simulink model "PiSimulink_MCU"  (R2020b)
settings: Solver=FixedStepDiscrete  StartTime=0.0  StopTime=10.0  FixedStep=0.001  RelTol=1e-3  EnableMultiTasking=on
InitFcn:
  | mbd_s32k_consistency_checks(bdroot(gcs));
undefined symbols (not defined in the file): LQFP
libraries: mbd_s32k1xx_ec_toolbox x13, simulink x2
(part 1 of 2)
Description:
  | This code is the MCU half of the Simulink on Raspberry Pi Guide.
  | It determines the data that is sent from the MCU.
  | 
  | Extra Modules (In addition to default functions):
  | LPSPI1 (Pi SPI logic moved from defaults to user area)
  | 
  | For more information, see our Simulink on Raspberry Pi Guide:
  | https://www.audesseinc.com/labs/resources/simulinkmpu/
  | 
  | Revision: 1.3
settings Model: LastModifiedBy=prasa
settings DataIOCC: ExternalInput=off  InitialState=off  SaveOutput=off  SignalLogging=off  SaveTime=off
settings OptimizationCC: DefaultParameterBehavior=Inlined  DefaultUnderspecifiedDataType=single  EnhancedBackFolding=on  PassReuseOutputArgsAs=Individual arguments  OptimizeBlockOrder=speed  EfficientTunableParamExpr=on
settings DebuggingCC: InheritedTsInSrcMsg=none  SingleTaskRateTransMsg=error  ParameterTunabilityLossMsg=error  UnconnectedInputMsg=error  UnconnectedOutputMsg=error  UnconnectedLineMsg=error  UnknownTsInhSupMsg=error  ArithmeticOperatorsInVariantConditions=warning
settings HardwareCC: ProdBitPerPointer=32  ProdBitPerSizeT=32  ProdBitPerPtrDiffT=32  ProdLargestAtomicInteger=Long  ProdLargestAtomicFloat=Double  ProdWordSize=32  ProdHWDeviceType=ARM Compatible->ARM Cortex
settings SFSimCC: MATLABDynamicMemAlloc=off  CustomCodeUndefinedFunction=UseInterfaceOnly
settings RTWCC: Description=Model Based Design Toolbox S32K1xx Code Generation Target  SystemTargetFile=mbd_s32k.tlc  MakeCommand=mbd_s32k_make_rtw COPY_MDLREF_INCLUDES=0  TemplateMakefile=mbd_s32k.tmf  GenerateReport=on  IncludeHyperlinkInReport=on  LaunchReport=on  GenerateTraceInfo=on  GenerateTraceReport=on  GenerateTraceReportSl=on  GenerateTraceReportSf=on  GenerateTraceReportEml=on
settings CodeAppCC: ForceParamTrailComments=on  IgnoreCustomStorageClasses=off  OperatorAnnotations=on  SimulinkDataObjDesc=on  SFDataObjDesc=on  InsertBlockDesc=on  StateflowObjectComments=on
settings STFCustomTargetCC: TargetLangStandard=C99 (ISO)  MultiwordLength=256  ConcurrentExecutionCompliant=off  CombineOutputUpdateFcns=on  ERTCustomFileBanners=on  SupportContinuousTime=off  SupportNonInlinedSFcns=off  RemoveResetFunc=on  MATLABClassNameForMDSCustomization=Simulink.SoftwareTarget.ERTCustomization  CPPClassGenCompliant=off  GRTInterface=off  SystemTargetFile=mbd_s32k.tlc
settings ERTTargetCC: TargetLangStandard=C99 (ISO)  ParMdlRefBuildCompliant=off  CompOptLevelCompliant=off  ConcurrentExecutionCompliant=off  ModelStepFunctionPrototypeControlCompliant=off  CPPClassGenCompliant=off  UseToolchainInfoCompliant=off  InlinedParameterPlacement=NonHierarchical  ERTSrcFileBannerTemplate=mbd_ert_code_template.cgt  ERTHdrFileBannerTemplate=mbd_ert_code_template.cgt  ERTDataSrcFileTemplate=mbd_ert_code_template.cgt  ERTDataHdrFileTemplate=mbd_ert_code_template.cgt  ERTCustomFileTemplate=example_file_process.tlc

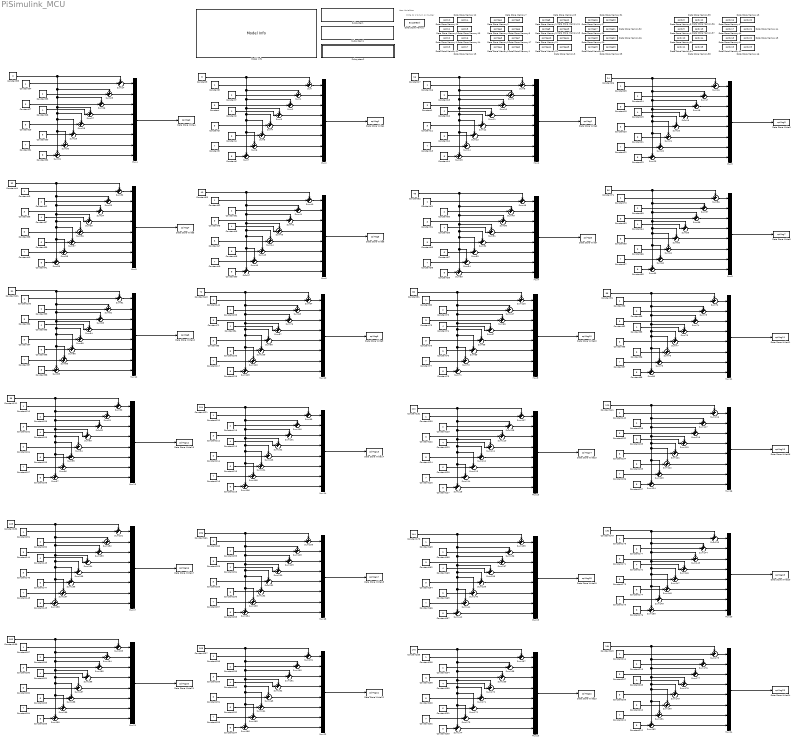
== system PiSimulink_MCU ==
  note: User Variables
  note: Write to 1 to turn on buzzer
  Constant{,1,18,27,36,45,54,63,72..73,82,92,102,112,122,132,144,153,162,171,180,189,198,207} (24 alike) : Constant  Value=3  OutDataTypeStr=uint8
  Constant{2,10,19,28,37,46,55,64,74,83..84,93,103,113,123,133,145,154,163,172,181,190,199,208} (24 alike) : Constant  Value=4  OutDataTypeStr=uint8
  Constant{8,16,25,34,43,52,61,70,80,90,100,110,120,130,140,142,151,160,169,178,187,196,205,214} (24 alike) : Constant  OutDataTypeStr=uint8
  Constant101 : Constant  Value=64  OutDataTypeStr=uint8
  Constant{3,11,20,29,38,47,56,65,75,85,94..95,104,114,124,134,146,155,164,173,182,191,200,209} (24 alike) : Constant  Value=5  OutDataTypeStr=uint8
  Constant{4,12,21,30,39,48,57,66,76,86,96,105..106,115,125,135,147,156,165,174,183,192,201,210} (24 alike) : Constant  Value=6  OutDataTypeStr=uint8
  Constant{5,13,22,31,40,49,58,67,77,87,97,107,116..117,126,136,148,157,166,175,184,193,202,211} (24 alike) : Constant  Value=7  OutDataTypeStr=uint8
  Constant{6,9,14,23,32,41,50,59,68,78,88,98,108,118,127..128,137,149,158,167,176,185,194,203,212} (25 alike) : Constant  Value=8  OutDataTypeStr=uint8
  Constant{7,15,24,33,42,51,60,69,79,89,99,109,119,129,138..139,150,159,168,177,186,195,204,213} (24 alike) : Constant  Value=2  OutDataTypeStr=uint8
  Constant111 : Constant  Value=96  OutDataTypeStr=uint8
  Constant121 : Constant  Value=104  OutDataTypeStr=uint8
  Constant131 : Constant  Value=112  OutDataTypeStr=uint8
  Constant141 : Constant  Value=120  OutDataTypeStr=uint8
  Constant143 : Constant  Value=72  OutDataTypeStr=uint8
  Constant152 : Constant  Value=128  OutDataTypeStr=uint8
  Constant161 : Constant  Value=136  OutDataTypeStr=uint8
  Constant17 : Constant  Value=16  OutDataTypeStr=uint8
  Constant170 : Constant  Value=144  OutDataTypeStr=uint8
  Constant179 : Constant  Value=152  OutDataTypeStr=uint8
  Constant188 : Constant  Value=160  OutDataTypeStr=uint8
  Constant197 : Constant  Value=168  OutDataTypeStr=uint8
  Constant206 : Constant  Value=176  OutDataTypeStr=uint8
  Constant215 : Constant  Value=184  OutDataTypeStr=uint8
  Constant26 : Constant  Value=24  OutDataTypeStr=uint8
  Constant35 : Constant  Value=0  OutDataTypeStr=uint8
  Constant44 : Constant  Value=32  OutDataTypeStr=uint8
  Constant53 : Constant  Value=40  OutDataTypeStr=uint8
  Constant62 : Constant  Value=48  OutDataTypeStr=uint8
  Constant71 : Constant  Value=56  OutDataTypeStr=uint8
  Constant81 : Constant  Value=80  OutDataTypeStr=uint8
  Constant91 : Constant  Value=88  OutDataTypeStr=uint8
  Data Store Memory : DataStoreMemory  DataStoreName=BuzzerBool  ReadBeforeWriteMsg=warning  WriteAfterWriteMsg=warning  WriteAfterReadMsg=warning  ShowAdditionalParam=off  OutDataTypeStr=boolean
  Data Store Memory1 : DataStoreMemory  DataStoreName=spiMsg0  ReadBeforeWriteMsg=warning  WriteAfterWriteMsg=warning  WriteAfterReadMsg=warning  InitialValue=[255 255 255 255 255 255 255 255]  ShowAdditionalParam=off  OutDataTypeStr=uint8
  Data Store Memory10 : DataStoreMemory  DataStoreName=spiRx2  ReadBeforeWriteMsg=warning  WriteAfterWriteMsg=warning  WriteAfterReadMsg=warning  InitialValue=[255 255 255 255 255 255 255 255]  ShowAdditionalParam=off  OutDataTypeStr=uint8
  Data Store Memory11 : DataStoreMemory  DataStoreName=spiRx3  ReadBeforeWriteMsg=warning  WriteAfterWriteMsg=warning  WriteAfterReadMsg=warning  InitialValue=[255 255 255 255 255 255 255 255]  ShowAdditionalParam=off  OutDataTypeStr=uint8
  Data Store Memory12 : DataStoreMemory  DataStoreName=spiRx4  ReadBeforeWriteMsg=warning  WriteAfterWriteMsg=warning  WriteAfterReadMsg=warning  InitialValue=[255 255 255 255 255 255 255 255]  ShowAdditionalParam=off  OutDataTypeStr=uint8
  Data Store Memory13 : DataStoreMemory  DataStoreName=spiRx5  ReadBeforeWriteMsg=warning  WriteAfterWriteMsg=warning  WriteAfterReadMsg=warning  InitialValue=[255 255 255 255 255 255 255 255]  ShowAdditionalParam=off  OutDataTypeStr=uint8
  Data Store Memory14 : DataStoreMemory  DataStoreName=spiRx6  ReadBeforeWriteMsg=warning  WriteAfterWriteMsg=warning  WriteAfterReadMsg=warning  InitialValue=[255 255 255 255 255 255 255 255]  ShowAdditionalParam=off  OutDataTypeStr=uint8
  Data Store Memory15 : DataStoreMemory  DataStoreName=spiRx7  ReadBeforeWriteMsg=warning  WriteAfterWriteMsg=warning  WriteAfterReadMsg=warning  InitialValue=[255 255 255 255 255 255 255 255]  ShowAdditionalParam=off  OutDataTypeStr=uint8
  Data Store Memory16 : DataStoreMemory  DataStoreName=spiRx0  ReadBeforeWriteMsg=warning  WriteAfterWriteMsg=warning  WriteAfterReadMsg=warning  InitialValue=[255 255 255 255 255 255 255 255]  ShowAdditionalParam=off  OutDataTypeStr=uint8
  Data Store Memory17 : DataStoreMemory  DataStoreName=spiMsg7  ReadBeforeWriteMsg=warning  WriteAfterWriteMsg=warning  WriteAfterReadMsg=warning  InitialValue=[255 255 255 255 255 255 255 255]  ShowAdditionalParam=off  OutDataTypeStr=uint8
  Data Store Memory18 : DataStoreMemory  DataStoreName=spiMsg14  ReadBeforeWriteMsg=warning  WriteAfterWriteMsg=warning  WriteAfterReadMsg=warning  InitialValue=[255 255 255 255 255 255 255 255]  ShowAdditionalParam=off  OutDataTypeStr=uint8
  Data Store Memory19 : DataStoreMemory  DataStoreName=spiMsg8  ReadBeforeWriteMsg=warning  WriteAfterWriteMsg=warning  WriteAfterReadMsg=warning  InitialValue=[255 255 255 255 255 255 255 255]  ShowAdditionalParam=off  OutDataTypeStr=uint8
  Data Store Memory2 : DataStoreMemory  DataStoreName=spiMsg1  ReadBeforeWriteMsg=warning  WriteAfterWriteMsg=warning  WriteAfterReadMsg=warning  InitialValue=[255 255 255 255 255 255 255 255]  ShowAdditionalParam=off  OutDataTypeStr=uint8
  Data Store Memory20 : DataStoreMemory  DataStoreName=spiMsg9  ReadBeforeWriteMsg=warning  WriteAfterWriteMsg=warning  WriteAfterReadMsg=warning  InitialValue=[255 255 255 255 255 255 255 255]  ShowAdditionalParam=off  OutDataTypeStr=uint8
  Data Store Memory21 : DataStoreMemory  DataStoreName=spiMsg10  ReadBeforeWriteMsg=warning  WriteAfterWriteMsg=warning  WriteAfterReadMsg=warning  InitialValue=[255 255 255 255 255 255 255 255]  ShowAdditionalParam=off  OutDataTypeStr=uint8
  Data Store Memory22 : DataStoreMemory  DataStoreName=spiMsg11  ReadBeforeWriteMsg=warning  WriteAfterWriteMsg=warning  WriteAfterReadMsg=warning  InitialValue=[255 255 255 255 255 255 255 255]  ShowAdditionalParam=off  OutDataTypeStr=uint8
  Data Store Memory23 : DataStoreMemory  DataStoreName=spiMsg12  ReadBeforeWriteMsg=warning  WriteAfterWriteMsg=warning  WriteAfterReadMsg=warning  InitialValue=[255 255 255 255 255 255 255 255]  ShowAdditionalParam=off  OutDataTypeStr=uint8
  Data Store Memory24 : DataStoreMemory  DataStoreName=spiMsg13  ReadBeforeWriteMsg=warning  WriteAfterWriteMsg=warning  WriteAfterReadMsg=warning  InitialValue=[255 255 255 255 255 255 255 255]  ShowAdditionalParam=off  OutDataTypeStr=uint8
  Data Store Memory25 : DataStoreMemory  DataStoreName=spiMsg23  ReadBeforeWriteMsg=warning  WriteAfterWriteMsg=warning  WriteAfterReadMsg=warning  InitialValue=[255 255 255 255 255 255 255 255]  ShowAdditionalParam=off  OutDataTypeStr=uint8
  Data Store Memory26 : DataStoreMemory  DataStoreName=spiMsg22  ReadBeforeWriteMsg=warning  WriteAfterWriteMsg=warning  WriteAfterReadMsg=warning  InitialValue=[255 255 255 255 255 255 255 255]  ShowAdditionalParam=off  OutDataTypeStr=uint8
  Data Store Memory27 : DataStoreMemory  DataStoreName=spiMsg16  ReadBeforeWriteMsg=warning  WriteAfterWriteMsg=warning  WriteAfterReadMsg=warning  InitialValue=[255 255 255 255 255 255 255 255]  ShowAdditionalParam=off  OutDataTypeStr=uint8
  Data Store Memory28 : DataStoreMemory  DataStoreName=spiMsg17  ReadBeforeWriteMsg=warning  WriteAfterWriteMsg=warning  WriteAfterReadMsg=warning  InitialValue=[255 255 255 255 255 255 255 255]  ShowAdditionalParam=off  OutDataTypeStr=uint8
  Data Store Memory29 : DataStoreMemory  DataStoreName=spiMsg18  ReadBeforeWriteMsg=warning  WriteAfterWriteMsg=warning  WriteAfterReadMsg=warning  InitialValue=[255 255 255 255 255 255 255 255]  ShowAdditionalParam=off  OutDataTypeStr=uint8
  Data Store Memory3 : DataStoreMemory  DataStoreName=spiMsg15  ReadBeforeWriteMsg=warning  WriteAfterWriteMsg=warning  WriteAfterReadMsg=warning  InitialValue=[255 255 255 255 255 255 255 255]  ShowAdditionalParam=off  OutDataTypeStr=uint8
  Data Store Memory30 : DataStoreMemory  DataStoreName=spiMsg19  ReadBeforeWriteMsg=warning  WriteAfterWriteMsg=warning  WriteAfterReadMsg=warning  InitialValue=[255 255 255 255 255 255 255 255]  ShowAdditionalParam=off  OutDataTypeStr=uint8
  Data Store Memory31 : DataStoreMemory  DataStoreName=spiMsg20  ReadBeforeWriteMsg=warning  WriteAfterWriteMsg=warning  WriteAfterReadMsg=warning  InitialValue=[255 255 255 255 255 255 255 255]  ShowAdditionalParam=off  OutDataTypeStr=uint8
  Data Store Memory32 : DataStoreMemory  DataStoreName=spiMsg21  ReadBeforeWriteMsg=warning  WriteAfterWriteMsg=warning  WriteAfterReadMsg=warning  InitialValue=[255 255 255 255 255 255 255 255]  ShowAdditionalParam=off  OutDataTypeStr=uint8
  Data Store Memory33 : DataStoreMemory  DataStoreName=spiRx10  ReadBeforeWriteMsg=warning  WriteAfterWriteMsg=warning  WriteAfterReadMsg=warning  InitialValue=[255 255 255 255 255 255 255 255]  ShowAdditionalParam=off  OutDataTypeStr=uint8
  Data Store Memory34 : DataStoreMemory  DataStoreName=spiRx11  ReadBeforeWriteMsg=warning  WriteAfterWriteMsg=warning  WriteAfterReadMsg=warning  InitialValue=[255 255 255 255 255 255 255 255]  ShowAdditionalParam=off  OutDataTypeStr=uint8
  Data Store Memory35 : DataStoreMemory  DataStoreName=spiRx12  ReadBeforeWriteMsg=warning  WriteAfterWriteMsg=warning  WriteAfterReadMsg=warning  InitialValue=[255 255 255 255 255 255 255 255]  ShowAdditionalParam=off  OutDataTypeStr=uint8
  Data Store Memory36 : DataStoreMemory  DataStoreName=spiRx13  ReadBeforeWriteMsg=warning  WriteAfterWriteMsg=warning  WriteAfterReadMsg=warning  InitialValue=[255 255 255 255 255 255 255 255]  ShowAdditionalParam=off  OutDataTypeStr=uint8
  Data Store Memory37 : DataStoreMemory  DataStoreName=spiRx14  ReadBeforeWriteMsg=warning  WriteAfterWriteMsg=warning  WriteAfterReadMsg=warning  InitialValue=[255 255 255 255 255 255 255 255]  ShowAdditionalParam=off  OutDataTypeStr=uint8
  Data Store Memory38 : DataStoreMemory  DataStoreName=spiRx15  ReadBeforeWriteMsg=warning  WriteAfterWriteMsg=warning  WriteAfterReadMsg=warning  InitialValue=[255 255 255 255 255 255 255 255]  ShowAdditionalParam=off  OutDataTypeStr=uint8
  Data Store Memory39 : DataStoreMemory  DataStoreName=spiRx8  ReadBeforeWriteMsg=warning  WriteAfterWriteMsg=warning  WriteAfterReadMsg=warning  InitialValue=[255 255 255 255 255 255 255 255]  ShowAdditionalParam=off  OutDataTypeStr=uint8
  Data Store Memory4 : DataStoreMemory  DataStoreName=spiMsg2  ReadBeforeWriteMsg=warning  WriteAfterWriteMsg=warning  WriteAfterReadMsg=warning  InitialValue=[255 255 255 255 255 255 255 255]  ShowAdditionalParam=off  OutDataTypeStr=uint8
  Data Store Memory40 : DataStoreMemory  DataStoreName=spiRx9  ReadBeforeWriteMsg=warning  WriteAfterWriteMsg=warning  WriteAfterReadMsg=warning  InitialValue=[255 255 255 255 255 255 255 255]  ShowAdditionalParam=off  OutDataTypeStr=uint8
  Data Store Memory41 : DataStoreMemory  DataStoreName=spiRx18  ReadBeforeWriteMsg=warning  WriteAfterWriteMsg=warning  WriteAfterReadMsg=warning  InitialValue=[255 255 255 255 255 255 255 255]  ShowAdditionalParam=off  OutDataTypeStr=uint8
  Data Store Memory42 : DataStoreMemory  DataStoreName=spiRx19  ReadBeforeWriteMsg=warning  WriteAfterWriteMsg=warning  WriteAfterReadMsg=warning  InitialValue=[255 255 255 255 255 255 255 255]  ShowAdditionalParam=off  OutDataTypeStr=uint8
  Data Store Memory43 : DataStoreMemory  DataStoreName=spiRx20  ReadBeforeWriteMsg=warning  WriteAfterWriteMsg=warning  WriteAfterReadMsg=warning  InitialValue=[255 255 255 255 255 255 255 255]  ShowAdditionalParam=off  OutDataTypeStr=uint8
  Data Store Memory44 : DataStoreMemory  DataStoreName=spiRx21  ReadBeforeWriteMsg=warning  WriteAfterWriteMsg=warning  WriteAfterReadMsg=warning  InitialValue=[255 255 255 255 255 255 255 255]  ShowAdditionalParam=off  OutDataTypeStr=uint8
  Data Store Memory45 : DataStoreMemory  DataStoreName=spiRx22  ReadBeforeWriteMsg=warning  WriteAfterWriteMsg=warning  WriteAfterReadMsg=warning  InitialValue=[255 255 255 255 255 255 255 255]  ShowAdditionalParam=off  OutDataTypeStr=uint8
  Data Store Memory46 : DataStoreMemory  DataStoreName=spiRx23  ReadBeforeWriteMsg=warning  WriteAfterWriteMsg=warning  WriteAfterReadMsg=warning  InitialValue=[255 255 255 255 255 255 255 255]  ShowAdditionalParam=off  OutDataTypeStr=uint8
  Data Store Memory47 : DataStoreMemory  DataStoreName=spiRx16  ReadBeforeWriteMsg=warning  WriteAfterWriteMsg=warning  WriteAfterReadMsg=warning  InitialValue=[255 255 255 255 255 255 255 255]  ShowAdditionalParam=off  OutDataTypeStr=uint8
  Data Store Memory48 : DataStoreMemory  DataStoreName=spiRx17  ReadBeforeWriteMsg=warning  WriteAfterWriteMsg=warning  WriteAfterReadMsg=warning  InitialValue=[255 255 255 255 255 255 255 255]  ShowAdditionalParam=off  OutDataTypeStr=uint8
  Data Store Memory5 : DataStoreMemory  DataStoreName=spiMsg3  ReadBeforeWriteMsg=warning  WriteAfterWriteMsg=warning  WriteAfterReadMsg=warning  InitialValue=[255 255 255 255 255 255 255 255]  ShowAdditionalParam=off  OutDataTypeStr=uint8
  Data Store Memory6 : DataStoreMemory  DataStoreName=spiMsg4  ReadBeforeWriteMsg=warning  WriteAfterWriteMsg=warning  WriteAfterReadMsg=warning  InitialValue=[255 255 255 255 255 255 255 255]  ShowAdditionalParam=off  OutDataTypeStr=uint8
  Data Store Memory7 : DataStoreMemory  DataStoreName=spiMsg5  ReadBeforeWriteMsg=warning  WriteAfterWriteMsg=warning  WriteAfterReadMsg=warning  InitialValue=[255 255 255 255 255 255 255 255]  ShowAdditionalParam=off  OutDataTypeStr=uint8
  Data Store Memory8 : DataStoreMemory  DataStoreName=spiMsg6  ReadBeforeWriteMsg=warning  WriteAfterWriteMsg=warning  WriteAfterReadMsg=warning  InitialValue=[255 255 255 255 255 255 255 255]  ShowAdditionalParam=off  OutDataTypeStr=uint8
  Data Store Memory9 : DataStoreMemory  DataStoreName=spiRx1  ReadBeforeWriteMsg=warning  WriteAfterWriteMsg=warning  WriteAfterReadMsg=warning  InitialValue=[255 255 255 255 255 255 255 255]  ShowAdditionalParam=off  OutDataTypeStr=uint8
  Data Store Write1 : DataStoreWrite  DataStoreName=spiMsg1
  Data Store Write10 : DataStoreWrite  DataStoreName=spiMsg10
  Data Store Write11 : DataStoreWrite  DataStoreName=spiMsg11
  Data Store Write12 : DataStoreWrite  DataStoreName=spiMsg8
  Data Store Write13 : DataStoreWrite  DataStoreName=spiMsg12
  Data Store Write14 : DataStoreWrite  DataStoreName=spiMsg13
  Data Store Write15 : DataStoreWrite  DataStoreName=spiMsg14
  Data Store Write16 : DataStoreWrite  DataStoreName=spiMsg15
  Data Store Write17 : DataStoreWrite  DataStoreName=spiMsg16
  Data Store Write18 : DataStoreWrite  DataStoreName=spiMsg17
  Data Store Write19 : DataStoreWrite  DataStoreName=spiMsg18
  Data Store Write2 : DataStoreWrite  DataStoreName=spiMsg2
  Data Store Write20 : DataStoreWrite  DataStoreName=spiMsg19
  Data Store Write21 : DataStoreWrite  DataStoreName=spiMsg20
  Data Store Write22 : DataStoreWrite  DataStoreName=spiMsg21
  Data Store Write23 : DataStoreWrite  DataStoreName=spiMsg22
  Data Store Write24 : DataStoreWrite  DataStoreName=spiMsg23
  Data Store Write3 : DataStoreWrite  DataStoreName=spiMsg3
  Data Store Write4 : DataStoreWrite  DataStoreName=spiMsg0
  Data Store Write5 : DataStoreWrite  DataStoreName=spiMsg4
  Data Store Write6 : DataStoreWrite  DataStoreName=spiMsg5
  Data Store Write7 : DataStoreWrite  DataStoreName=spiMsg6
  Data Store Write8 : DataStoreWrite  DataStoreName=spiMsg7
  Data Store Write9 : DataStoreWrite  DataStoreName=spiMsg9
  Model Info : simulink/Model-Wide Utilities/Model Info  Frame=on  DisplayStringWithTags=|  HorizontalTextAlignment=Left  LeftAlignmentValue=0.02
      | Audesse Simulink Samples: %<ModelName>
      | 
      | %<Description>
  Mux{1..24} (24 alike) : Mux  Inputs=8
  Subsystem : Subsystem  Priority=1
      mask Display:
      | scl=1/4;
      | patch(scl*[0,52,90,54],scl*[16,55,146,146],[16/255,118/255,188/255],'bottom-left');
      | patch(scl*[0,27,82,77,68],scl*[16,0,42,62,69],[46/255,49/255,146/255],'bottom-left');
      | patch(scl*[89,125,90,68],scl*[16,16,146,91],[0,0,0],'bottom-left');
      | disp('Hardware Modules Config\n(SPI,CAN,ADC,etc..)');
  Subsystem1 : Subsystem
      mask Display:
      | scl=1/4;
      | patch(scl*[0,52,90,54],scl*[16,55,146,146],[16/255,118/255,188/255],'bottom-left');
      | patch(scl*[0,27,82,77,68],scl*[16,0,42,62,69],[46/255,49/255,146/255],'bottom-left');
      | patch(scl*[89,125,90,68],scl*[16,16,146,91],[0,0,0],'bottom-left');
      | disp('Default Control Functions\n(Do not modify unless you know what you are doing)');
  Subsystem2 : Subsystem
      mask Display:
      | scl=1/4;
      | patch(scl*[0,52,90,54],scl*[16,55,146,146],[16/255,118/255,188/255],'bottom-left');
      | patch(scl*[0,27,82,77,68],scl*[16,0,42,62,69],[46/255,49/255,146/255],'bottom-left');
      | patch(scl*[89,125,90,68],scl*[16,16,146,91],[0,0,0],'bottom-left');
      | disp('Run Once at Startup');
  Sum{,1..191} (192 alike) : Sum  Inputs=++|
  wires:
  Mux2/1 -> Data Store Write1/1
  Sum/1 -> Mux2/1
  Sum1/1 -> Mux2/2
  Sum2/1 -> Mux2/3
  Sum3/1 -> Mux2/4
  Sum4/1 -> Mux2/5
  Sum7/1 -> Mux2/8
  Sum6/1 -> Mux2/7
  Sum5/1 -> Mux2/6
  Constant6/1 -> Sum7/2
  Constant5/1 -> Sum6/2
  Constant4/1 -> Sum5/2
  Constant3/1 -> Sum4/2
  Constant2/1 -> Sum3/2
  Constant/1 -> Sum2/2
  Constant7/1 -> Sum1/2
  Constant8/1 -> Sum/2
  Constant9/1 -> Sum1/1, Sum2/1, Sum3/1, Sum4/1, Sum7/1, Sum6/1, Sum5/1, Sum/1
  Sum9/1 -> Mux1/2
  Sum8/1 -> Mux1/1
  Sum14/1 -> Mux1/7
  Constant15/1 -> Sum9/2
  Constant11/1 -> Sum12/2
  Constant10/1 -> Sum11/2
  Constant12/1 -> Sum13/2
  Constant16/1 -> Sum8/2
  Sum10/1 -> Mux1/3
  Sum11/1 -> Mux1/4
  Sum13/1 -> Mux1/6
  Constant14/1 -> Sum15/2
  Sum15/1 -> Mux1/8
  Mux1/1 -> Data Store Write2/1
  Constant17/1 -> Sum9/1, Sum10/1, Sum11/1, Sum12/1, Sum15/1, Sum14/1, Sum13/1, Sum8/1
  Constant1/1 -> Sum10/2
  Sum12/1 -> Mux1/5
  Constant13/1 -> Sum14/2
  Sum17/1 -> Mux3/2
  Sum16/1 -> Mux3/1
  Sum22/1 -> Mux3/7
  Constant24/1 -> Sum17/2
  Constant20/1 -> Sum20/2
  Constant19/1 -> Sum19/2
  Constant21/1 -> Sum21/2
  Constant25/1 -> Sum16/2
  Sum18/1 -> Mux3/3
  Sum19/1 -> Mux3/4
  Sum21/1 -> Mux3/6
  Constant23/1 -> Sum23/2
  Sum23/1 -> Mux3/8
  Mux3/1 -> Data Store Write3/1
  Constant26/1 -> Sum17/1, Sum18/1, Sum19/1, Sum20/1, Sum23/1, Sum22/1, Sum21/1, Sum16/1
  Constant18/1 -> Sum18/2
  Sum20/1 -> Mux3/5
  Constant22/1 -> Sum22/2
  Sum25/1 -> Mux4/2
  Sum24/1 -> Mux4/1
  Sum30/1 -> Mux4/7
  Constant33/1 -> Sum25/2
  Constant29/1 -> Sum28/2
  Constant28/1 -> Sum27/2
  Constant30/1 -> Sum29/2
  Constant34/1 -> Sum24/2
  Sum26/1 -> Mux4/3
  Sum27/1 -> Mux4/4
  Sum29/1 -> Mux4/6
  Constant32/1 -> Sum31/2
  Sum31/1 -> Mux4/8
  Mux4/1 -> Data Store Write4/1
  Constant35/1 -> Sum25/1, Sum26/1, Sum27/1, Sum28/1, Sum31/1, Sum30/1, Sum29/1, Sum24/1
  Constant27/1 -> Sum26/2
  Sum28/1 -> Mux4/5
  Constant31/1 -> Sum30/2
  Sum33/1 -> Mux5/2
  Sum32/1 -> Mux5/1
  Sum38/1 -> Mux5/7
  Constant42/1 -> Sum33/2
  Constant38/1 -> Sum36/2
  Constant37/1 -> Sum35/2
  Constant39/1 -> Sum37/2
  Constant43/1 -> Sum32/2
  Sum34/1 -> Mux5/3
  Sum35/1 -> Mux5/4
  Sum37/1 -> Mux5/6
  Constant41/1 -> Sum39/2
  Sum39/1 -> Mux5/8
  Mux5/1 -> Data Store Write5/1
  Constant44/1 -> Sum33/1, Sum34/1, Sum35/1, Sum36/1, Sum39/1, Sum38/1, Sum37/1, Sum32/1
  Constant36/1 -> Sum34/2
  Sum36/1 -> Mux5/5
  Constant40/1 -> Sum38/2
  Sum41/1 -> Mux6/2
  Sum40/1 -> Mux6/1
  Sum46/1 -> Mux6/7
  Constant51/1 -> Sum41/2
  Constant47/1 -> Sum44/2
  Constant46/1 -> Sum43/2
  Constant48/1 -> Sum45/2
  Constant52/1 -> Sum40/2
  Sum42/1 -> Mux6/3
  Sum43/1 -> Mux6/4
  Sum45/1 -> Mux6/6
  Constant50/1 -> Sum47/2
  Sum47/1 -> Mux6/8
  Mux6/1 -> Data Store Write6/1
  Constant53/1 -> Sum41/1, Sum42/1, Sum43/1, Sum44/1, Sum47/1, Sum46/1, Sum45/1, Sum40/1
  Constant45/1 -> Sum42/2
  Sum44/1 -> Mux6/5
  Constant49/1 -> Sum46/2
  Sum49/1 -> Mux7/2
  Sum48/1 -> Mux7/1
  Sum54/1 -> Mux7/7
  Constant60/1 -> Sum49/2
  Constant56/1 -> Sum52/2
  Constant55/1 -> Sum51/2
  Constant57/1 -> Sum53/2
  Constant61/1 -> Sum48/2
  Sum50/1 -> Mux7/3
  Sum51/1 -> Mux7/4
  Sum53/1 -> Mux7/6
  Constant59/1 -> Sum55/2
  Sum55/1 -> Mux7/8
  Mux7/1 -> Data Store Write7/1
  Constant62/1 -> Sum49/1, Sum50/1, Sum51/1, Sum52/1, Sum55/1, Sum54/1, Sum53/1, Sum48/1
  Constant54/1 -> Sum50/2
  Sum52/1 -> Mux7/5
  Constant58/1 -> Sum54/2
  Sum57/1 -> Mux8/2
  Sum56/1 -> Mux8/1
  Sum62/1 -> Mux8/7
  Constant69/1 -> Sum57/2
  Constant65/1 -> Sum60/2
  Constant64/1 -> Sum59/2
  Constant66/1 -> Sum61/2
  Constant70/1 -> Sum56/2
  Sum58/1 -> Mux8/3
  Sum59/1 -> Mux8/4
  Sum61/1 -> Mux8/6
  Constant68/1 -> Sum63/2
  Sum63/1 -> Mux8/8
  Mux8/1 -> Data Store Write8/1
  Constant71/1 -> Sum57/1, Sum58/1, Sum59/1, Sum60/1, Sum63/1, Sum62/1, Sum61/1, Sum56/1
  Constant63/1 -> Sum58/2
  Sum60/1 -> Mux8/5
  Constant67/1 -> Sum62/2
  Constant81/1 -> Sum127/1, Sum66/1, Sum67/1, Sum68/1, Sum71/1, Sum70/1, Sum69/1, Sum126/1
  Constant73/1 -> Sum66/2
  Sum66/1 -> Mux9/3
  Sum71/1 -> Mux9/8
  Sum67/1 -> Mux9/4
  Constant75/1 -> Sum68/2
  Sum126/1 -> Mux9/1
  Constant76/1 -> Sum69/2
  Constant111/1 -> Sum91/1, Sum92/1, Sum93/1, Sum94/1, Sum97/1, Sum96/1, Sum95/1, Sum90/1
  Constant102/1 -> Sum92/2
  Sum94/1 -> Mux13/5
  Mux13/1 -> Data Store Write13/1
  Sum70/1 -> Mux9/7
  Sum97/1 -> Mux13/8
  Sum93/1 -> Mux13/4
  Constant105/1 -> Sum95/2
  Constant110/1 -> Sum90/2
  Constant103/1 -> Sum93/2
  Sum91/1 -> Mux13/2
  Sum96/1 -> Mux13/7
  Sum90/1 -> Mux13/1
  Constant109/1 -> Sum91/2
  Sum65/1 -> Mux10/2
  Constant133/1 -> Sum119/2
  Constant135/1 -> Sum122/2
  Constant134/1 -> Sum121/2
  Sum116/1 -> Mux16/1
  Constant138/1 -> Sum117/2
  Sum123/1 -> Mux16/7
  Sum117/1 -> Mux16/2
  Constant126/1 -> Sum114/2
  Constant136/1 -> Sum123/2
  Constant122/1 -> Sum110/2
  Constant79/1 -> Sum127/2
  Sum111/1 -> Mux15/4
  Sum121/1 -> Mux16/5
  Constant132/1 -> Sum118/2
  Sum115/1 -> Mux15/8
  Sum113/1 -> Mux15/6
  Constant127/1 -> Sum115/2
  Constant129/1 -> Sum108/2
  Sum107/1 -> Mux15/1
  Constant125/1 -> Sum113/2
  Constant124/1 -> Sum112/2
  Constant141/1 -> Sum117/1, Sum118/1, Sum119/1, Sum121/1, Sum124/1, Sum123/1, Sum122/1, Sum116/1
  Constant77/1 -> Sum70/2
  Sum114/1 -> Mux15/7
  Constant123/1 -> Sum111/2
  Sum68/1 -> Mux9/5
  Sum108/1 -> Mux15/2
  Mux16/1 -> Data Store Write16/1
  Constant104/1 -> Sum94/2
  Sum124/1 -> Mux16/8
  Constant137/1 -> Sum124/2
  Constant140/1 -> Sum116/2
  Sum118/1 -> Mux16/3
  Constant108/1 -> Sum97/2
  Sum119/1 -> Mux16/4
  Sum95/1 -> Mux13/6
  Sum73/1 -> Mux11/2
  Sum64/1 -> Mux10/1
  Constant116/1 -> Sum105/2
  Sum103/1 -> Mux14/5
  Sum92/1 -> Mux13/3
  Sum122/1 -> Mux16/6
  Constant121/1 -> Sum100/1, Sum101/1, Sum102/1, Sum103/1, Sum106/1, Sum105/1, Sum104/1, Sum99/1
  Constant112/1 -> Sum101/2
  Sum106/1 -> Mux14/8
  Constant118/1 -> Sum106/2
  Sum104/1 -> Mux14/6
  Constant131/1 -> Sum108/1, Sum110/1, Sum111/1, Sum112/1, Sum115/1, Sum114/1, Sum113/1, Sum107/1
  Sum102/1 -> Mux14/4
  Mux14/1 -> Data Store Write14/1
  Constant115/1 -> Sum104/2
  Constant78/1 -> Sum71/2
  Constant119/1 -> Sum100/2
  Sum101/1 -> Mux14/3
  Constant107/1 -> Sum96/2
  Constant120/1 -> Sum99/2
  Sum105/1 -> Mux14/7
  Sum100/1 -> Mux14/2
  Constant114/1 -> Sum103/2
  Constant113/1 -> Sum102/2
  Sum99/1 -> Mux14/1
  Sum120/1 -> Mux10/7
  Constant139/1 -> Sum65/2
  Constant87/1 -> Sum79/2
  Constant82/1 -> Sum74/2
  Sum77/1 -> Mux11/5
  Constant91/1 -> Sum73/1, Sum74/1, Sum75/1, Sum77/1, Sum80/1, Sum79/1, Sum78/1, Sum72/1
  Constant80/1 -> Sum126/2
  Mux11/1 -> Data Store Write11/1
  Sum75/1 -> Mux11/4
  Sum78/1 -> Mux11/6
  Constant88/1 -> Sum80/2
  Constant90/1 -> Sum72/2
  Constant89/1 -> Sum73/2
  Constant86/1 -> Sum78/2
  Sum72/1 -> Mux11/1
  Sum79/1 -> Mux11/7
  Constant130/1 -> Sum107/2
  Constant95/1 -> Sum98/2
  Constant84/1 -> Sum87/2
  Sum76/1 -> Mux10/3
  Sum87/1 -> Mux10/4
  Sum80/1 -> Mux11/8
  Constant97/1 -> Sum88/2
  Constant92/1 -> Sum83/2
  Sum85/1 -> Mux12/5
  Constant101/1 -> Sum82/1, Sum83/1, Sum84/1, Sum85/1, Sum89/1, Sum88/1, Sum86/1, Sum81/1
  Sum109/1 -> Mux10/6
  Mux15/1 -> Data Store Write15/1
  Sum69/1 -> Mux9/6
  Constant85/1 -> Sum77/2
  Constant74/1 -> Sum67/2
  Constant142/1 -> Sum64/2
  Sum83/1 -> Mux12/3
  Sum74/1 -> Mux11/3
  Mux12/1 -> Data Store Write12/1
  Sum86/1 -> Mux12/6
  Sum89/1 -> Mux12/8
  Constant93/1 -> Sum84/2
  Sum81/1 -> Mux12/1
  Constant96/1 -> Sum86/2
  Sum110/1 -> Mux15/3
  Constant106/1 -> Sum109/2
  Sum88/1 -> Mux12/7
  Constant99/1 -> Sum82/2
  Constant94/1 -> Sum85/2
  Sum112/1 -> Mux15/5
  Constant100/1 -> Sum81/2
  Constant83/1 -> Sum75/2
  Constant128/1 -> Sum125/2
  Sum84/1 -> Mux12/4
  Sum125/1 -> Mux10/8
  Sum127/1 -> Mux9/2
  Mux10/1 -> Data Store Write9/1
  Constant143/1 -> Sum65/1, Sum76/1, Sum87/1, Sum98/1, Sum125/1, Sum120/1, Sum109/1, Sum64/1
  Constant98/1 -> Sum89/2
  Mux9/1 -> Data Store Write10/1
  Sum82/1 -> Mux12/2
  Constant72/1 -> Sum76/2
  Sum98/1 -> Mux10/5
  Constant117/1 -> Sum120/2
  Constant164/1 -> Sum139/2
  Sum135/1 -> Mux19/1
  Constant165/1 -> Sum140/2
  Constant167/1 -> Sum142/2
  Sum140/1 -> Mux19/6
  Sum142/1 -> Mux19/8
  Constant171/1 -> Sum145/2
  Constant175/1 -> Sum149/2
  Constant162/1 -> Sum137/2
  Sum138/1 -> Mux19/4
  Sum147/1 -> Mux20/5
  Constant172/1 -> Sum146/2
  Sum149/1 -> Mux20/7
  Sum144/1 -> Mux20/2
  Sum143/1 -> Mux20/1
  Constant177/1 -> Sum144/2
  Constant173/1 -> Sum147/2
  Constant174/1 -> Sum148/2
  Constant166/1 -> Sum141/2
  Sum151/1 -> Mux17/1
  Constant150/1 -> Sum152/2
  Constant147/1 -> Sum156/2
  Constant151/1 -> Sum151/2
  Sum158/1 -> Mux17/8
  Sum157/1 -> Mux17/7
  Sum152/1 -> Mux17/2
  Constant168/1 -> Sum136/2
  Constant145/1 -> Sum154/2
  Mux17/1 -> Data Store Write17/1
  Sum155/1 -> Mux17/5
  Constant144/1 -> Sum153/2
  Constant152/1 -> Sum152/1, Sum153/1, Sum154/1, Sum155/1, Sum158/1, Sum157/1, Sum156/1, Sum151/1
  Constant158/1 -> Sum134/2
  Constant153/1 -> Sum129/2
  Sum132/1 -> Mux18/6
  Sum131/1 -> Mux18/5
  Constant157/1 -> Sum133/2
  Constant176/1 -> Sum150/2
  Sum150/1 -> Mux20/8
  Sum148/1 -> Mux20/6
  Sum136/1 -> Mux19/2
  Sum153/1 -> Mux17/3
  Sum141/1 -> Mux19/7
  Constant146/1 -> Sum155/2
  Constant161/1 -> Sum128/1, Sum129/1, Sum130/1, Sum131/1, Sum134/1, Sum133/1, Sum132/1, Sum159/1
  Mux20/1 -> Data Store Write20/1
  Sum145/1 -> Mux20/3
  Constant179/1 -> Sum144/1, Sum145/1, Sum146/1, Sum147/1, Sum150/1, Sum149/1, Sum148/1, Sum143/1
  Constant178/1 -> Sum143/2
  Sum156/1 -> Mux17/6
  Sum130/1 -> Mux18/4
  Mux18/1 -> Data Store Write18/1
  Constant156/1 -> Sum132/2
  Constant163/1 -> Sum138/2
  Sum154/1 -> Mux17/4
  Constant149/1 -> Sum158/2
  Sum139/1 -> Mux19/5
  Sum146/1 -> Mux20/4
  Sum137/1 -> Mux19/3
  Mux19/1 -> Data Store Write19/1
  Constant169/1 -> Sum135/2
  Sum159/1 -> Mux18/1
  Constant148/1 -> Sum157/2
  Sum129/1 -> Mux18/3
  Constant170/1 -> Sum136/1, Sum137/1, Sum138/1, Sum139/1, Sum142/1, Sum141/1, Sum140/1, Sum135/1
  Sum128/1 -> Mux18/2
  Constant159/1 -> Sum128/2
  Sum134/1 -> Mux18/8
  Constant160/1 -> Sum159/2
  Constant154/1 -> Sum130/2
  Sum133/1 -> Mux18/7
  Constant155/1 -> Sum131/2
  Sum167/1 -> Mux23/1
  Constant196/1 -> Sum191/2
  Sum166/1 -> Mux22/8
  Sum165/1 -> Mux22/7
  Constant191/1 -> Sum163/2
  Constant195/1 -> Sum160/2
  Constant190/1 -> Sum162/2
  Sum160/1 -> Mux22/2
  Sum161/1 -> Mux22/3
  Sum178/1 -> Mux24/4
  Mux23/1 -> Data Store Write23/1
  Sum169/1 -> Mux23/3
  Constant205/1 -> Sum167/2
  Sum171/1 -> Mux23/5
  Constant185/1 -> Sum190/2
  Sum191/1 -> Mux22/1
  Constant200/1 -> Sum171/2
  Constant214/1 -> Sum175/2
  Sum186/1 -> Mux21/4
  Mux22/1 -> Data Store Write22/1
  Sum188/1 -> Mux21/6
  Constant192/1 -> Sum164/2
  Constant199/1 -> Sum170/2
  Sum162/1 -> Mux22/4
  Constant184/1 -> Sum189/2
  Constant215/1 -> Sum176/1, Sum177/1, Sum178/1, Sum179/1, Sum182/1, Sum181/1, Sum180/1, Sum175/1
  Constant206/1 -> Sum168/1, Sum169/1, Sum170/1, Sum171/1, Sum174/1, Sum173/1, Sum172/1, Sum167/1
  Sum177/1 -> Mux24/3
  Mux24/1 -> Data Store Write24/1
  Constant197/1 -> Sum160/1, Sum161/1, Sum162/1, Sum163/1, Sum166/1, Sum165/1, Sum164/1, Sum191/1
  Sum168/1 -> Mux23/2
  Sum180/1 -> Mux24/6
  Constant212/1 -> Sum182/2
  Constant189/1 -> Sum161/2
  Sum185/1 -> Mux21/3
  Constant194/1 -> Sum166/2
  Mux21/1 -> Data Store Write21/1
  Sum173/1 -> Mux23/7
  Constant181/1 -> Sum186/2
  Sum187/1 -> Mux21/5
  Constant180/1 -> Sum185/2
  Constant187/1 -> Sum183/2
  Constant183/1 -> Sum188/2
  Sum163/1 -> Mux22/5
  Constant186/1 -> Sum184/2
  Constant188/1 -> Sum184/1, Sum185/1, Sum186/1, Sum187/1, Sum190/1, Sum189/1, Sum188/1, Sum183/1
  Sum189/1 -> Mux21/7
  Constant202/1 -> Sum173/2
  Sum183/1 -> Mux21/1
  Sum164/1 -> Mux22/6
  Sum184/1 -> Mux21/2
  Sum190/1 -> Mux21/8
  Sum181/1 -> Mux24/7
  Constant182/1 -> Sum187/2
  Constant208/1 -> Sum178/2
  Constant213/1 -> Sum176/2
  Sum175/1 -> Mux24/1
  Sum176/1 -> Mux24/2
  Sum170/1 -> Mux23/4
  Constant210/1 -> Sum180/2
  Sum182/1 -> Mux24/8
  Constant209/1 -> Sum179/2
  Constant204/1 -> Sum168/2
  Constant193/1 -> Sum165/2
  Constant207/1 -> Sum177/2
  Sum179/1 -> Mux24/5
  Constant211/1 -> Sum181/2
  Sum174/1 -> Mux23/8
  Sum172/1 -> Mux23/6
  Constant198/1 -> Sum169/2
  Constant201/1 -> Sum172/2
  Constant203/1 -> Sum174/2

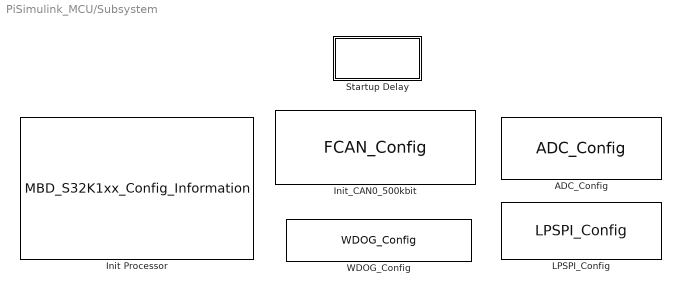
== system PiSimulink_MCU/Subsystem ==
  ADC_Config : mbd_s32k1xx_ec_toolbox/Motor Control Blocks/ADC Blocks/ADC_Config  instance=0  mode=12-bit conversion  smplts=20  adiclk=alternate clock 1  adiv=input clock  show_adv_opts=on  pretrgsel=PDB pre-trigger  swpretrg=Disabled  adtrg=software  trgsel=TRGMUX output  refsel=Vrefh and Vrefl  supply_monitoring=off  acfe=off  acfgt=off  acren=off  cv1=0  cv2=0  adco=off  avge=off  avgs=4 samples
  Init Processor : mbd_s32k1xx_ec_toolbox/MBD_S32K1xx_Config_Information  mbdt_ver=0  disp_str=|  config_params=[]  mcu_target_name=S32K144  mcu_target_package=100-LQFP  mcu_target_sram_size=64KB  mcu_system_clock_freq=80  mcu_xtal_freq=External 8  mcu_steptick_timer=LPIT Channel 0  mcu_steptick_prio=15  ds_import_enable=on  target_compiler=GCC  target_memory=FLASH  gcc_target_compile_opts=-mcpu=cortex-m4 -mthumb -mfloat-abi=hard -mfpu=fpv4-sp-d16 -O1 -g -gstrict-dwarf  gcc_target_assemble_opts=-mcpu=cortex-m4 -mthumb -mfloat-abi=hard -mfpu=fpv4-sp-d16 -g  gcc_target_link_opts=-mcpu=cortex-m4 -mthumb -mfloat-abi=hard -mfpu=fpv4-sp-d16  gcc_target_default_lcf=on  gcc_target_user_lcf=S32K148_192_flash.ld  ghs_target_compile_opts=-cpu=cortexm4f -thumb -DARM_MATH_CM4 -fpu=vfpv4_d16 -fsingle -Ogeneral -Wundef -Wimplicit-int -Wshadow -Wtrigraphs --no_commons --gnu_asm -gnu99 -gdwarf-2 -G  ghs_target_assemble_opts=-cpu=cortexm4f -fpu=vfpv4_d16  ghs_target_link_opts=-cpu=cortexm4f -thumb -fpu=vfpv4_d16  ghs_target_default_lcf=on  ghs_target_user_lcf=S32K148_192_flash.ld  iar_target_compile_opts=--cpu=Cortex-M4F --thumb --fpu=VFPv4_sp -Ol -e --debug --dlib_config normal  iar_target_assemble_opts=--cpu Cortex-M4F --thumb --fpu VFPv4_sp  iar_target_link_opts=--no_exceptions --vfe --inline  iar_target_default_lcf=on  iar_target_user_lcf=S32K148_192_flash.icf  pil_download_enable=off  rbl_download_enable=off  rbl_start_delay=5000000  rbl_download_interface=OpenSDA  rbl_restart_request=off  rbl_com_port=Custom  rbl_com_port_custom=COM1  pil_download_rate=57600  pil_opensda_drive=Custom  pil_opensda_drive_custom=D  pil_uart_instance=1  pil_uart_rx=PTC6: [LPUART1_RX | Receive]  pil_uart_tx=PTC7: [LPUART1_TX | Transmit]  FTM_PWM_PcrCheckEnDis=on  FTM_Input_Edge_Inputs_PcrCheckEnDis=on  FTM_Dual_Edge_Inputs_PcrCheckEnDis=on  FTM_Quadrature_Inputs_PcrCheckEnDis=on  FTM_Hall_Sensor_Inputs_PcrCheckEnDis=on  LPTMR_PcrCheckEnDis=on  PIT_PcrCheckEnDis=on  RTC_PcrCheckEnDis=on  FlexCAN_PcrCheckEnDis=on  LIN_PcrCheckEnDis=on  FlexIO_PcrCheckEnDis=on  LPI2C_PcrCheckEnDis=on  LPSPI_PcrCheckEnDis=on  LPUART_PcrCheckEnDis=on  CMP_PcrCheckEnDis=on  GPIO_OutputPcrCheckEnDis=on  GPIO_InputPcrCheckEnDis=on  SBC_PcrCheckEnDis=on  BMS_PcrCheckEnDis=on  AMMCLIB_PcrCheckEnDis=on  FM_PcrCheckEnDis=on  Profile_PcrCheckEnDis=on  ConfigParams_PcrCheckEnDis=on  ModelRef_PcrCheckEnDis=on  PDB0_PcrCheckEnDis=on  CSEc_PcrCheckEnDis=on  eDMA_PcrCheckEnDis=on  FLASH_PcrCheckEnDis=on  ADC_PcrCheckEnDis=on  WDOG_PcrCheckEnDis=on
      | Target : S32K144-64KB_SRAM
      | Package : 100-pin
      | System clock : 80 MHz
      | XTAL clock : External 8 MHz
      | Compiler : IAR
      | Target Type : FLASH
      | Download Code after build : off
      | Step Tick Interrupt Priority : 15
  Init_CAN0_500kbit : mbd_s32k1xx_ec_toolbox/Communication Blocks/CAN Blocks/FCAN_Config  can_instance=0  can_mode=Normal mode  can_max_num_mb=16  can_rx=PTB0: [CAN0_RX | CAN Rx channel]  can_tx=PTB1: [CAN0_TX | CAN Tx Channel]  show_adv_opts=off  can_clk_src=Peripheral clock  bitrate=500  bitrate_adv_opts=off  can_presdiv=7  can_rjw=3  can_pseg1=6  can_pseg2=3  can_propseg=7  can_cbt_presdiv=9  can_cbt_rjw=0  can_cbt_pseg1=3  can_cbt_pseg2=3  can_cbt_propseg=6  can_fd_enable=off  can_payload=8  can_rxfifo_enable=off  can_fifo_id_filter_extended=off  can_fifo_id_filter_remote=off  can_num_id_filters=8  can_fifo_id_format=A  can_fifo_id_filter={'0x0', '0x0', '0x0', '0x0', '0x0', '0x0', '0x0', '0x0'}  can_pn_enable=off  can_wakeup_match=off  can_wakeup_timeout=off  can_timeout_en=off  can_match_timeout=1  can_multiple_matches_en=off  can_num_matches=1  can_idfilter_extendedid=off  can_idfilter_remoteframe=off  can_idfilter_type=Match exact  can_idfilter_id1=0  can_idfilter_id2=0  can_payloadfilter_enable=on  can_payloadfilter_dlclow=0  can_payloadfilter_dlchigh=0  can_payloadfilter_type=Match exact  can_payloadfilter_payload1_b0=0  can_payloadfilter_payload1_b1=0  can_payloadfilter_payload1_b2=0  can_payloadfilter_payload1_b3=0  can_payloadfilter_payload1_b4=0  can_payloadfilter_payload1_b5=0  can_payloadfilter_payload1_b6=0  can_payloadfilter_payload1_b7=0  can_payloadfilter_payload2_b0=0  can_payloadfilter_payload2_b1=0  can_payloadfilter_payload2_b2=0  can_payloadfilter_payload2_b3=0  can_payloadfilter_payload2_b4=0  can_payloadfilter_payload2_b5=0  can_payloadfilter_payload2_b6=0  can_payloadfilter_payload2_b7=0
  "LPSPI_Config " : mbd_s32k1xx_ec_toolbox/Communication Blocks/SPI Blocks/LPSPI_Config   InstanceNumber=1  Role=Slave  BaudRate=10000  ShowAdvanced=on  sin=PTB15: [LPSPI1_SIN | LPSPI Serial Data Input]  sout=PTB16: [LPSPI1_SOUT | LPSPI Serial Data Output]  sck=PTB14: [LPSPI1_SCK | LPSPI Serial Clock I/O]  pcs0=None  pcs1=None  pcs2=None  pcs3=PTB17: [LPSPI1_PCS3 | Peripheral Chip Select 3]  CPHA=1  CPOL=0  BitOrder=MSB first  TransferSize=8  WhichPCS=0  PCSPol=ActiveLow  ContinuousTransfer=on
  Startup Delay : Subsystem  mask(System Start){ShowInLibBrowser=0}
      mask prompts: ShowInLibBrowser "Simulink:masks:CustCodeMaskParam1_MP"
      settings: CopyFcn=cccopyfcn(gcb)  OpenFcn=ccopenfcn('System Start Function')
      mask Help: eval('feval(''rtwprivate'',''rtwhelpview'',''rtw_sys_start_block'')');
      mask Display: disp('System\nStart');
  WDOG_Config : mbd_s32k1xx_ec_toolbox/Core and System Blocks/WDOG Blocks/WDOG_Config  clk_source=LPO clock  window_enable=off  window_value=1000.000 milliseconds  timeout_value=1000.000 milliseconds  prescaler_enable=on  update_enable=off  int_enable=off  show_adv_opts=on

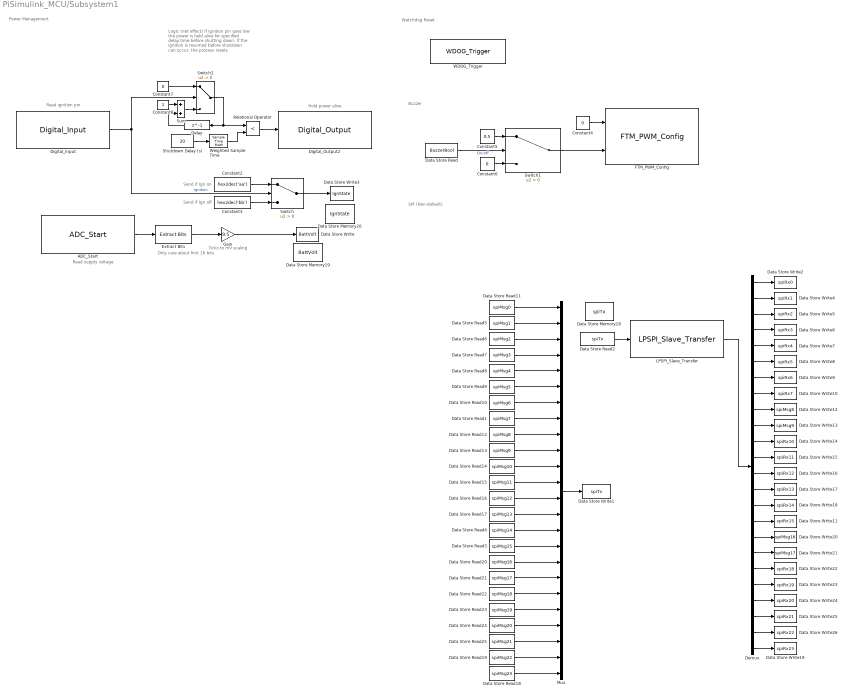
== system PiSimulink_MCU/Subsystem1 ==
  note: Watchdog Reset
  note: Power Management
  note: Read ignition pin
  note: Only care about
      | first 16 bits
  note: Ticks to mV scaling
  note: Read supply voltage
  note: Send if Ign on
  note: Send if Ign off
  note: SPI (Non-default)
  note: Buzzer
  note: Hold power alive
  note: Logic (net effect)
      | If ignition pin goes low the power is held alive for specified delay time before shutting down.
      |
      | If the ignition is resumed before shutdown can occur, the process resets
  ADC_Start : mbd_s32k1xx_ec_toolbox/Motor Control Blocks/ADC Blocks/ADC_Start  instance=0  adc_r=A  adc_chan=PTA6: [ADC0_SE2 | ADC Single Ended Input]  aien=off  mcuTargetUpdate=on
  Constant2 : Constant  Value=hex2dec('aa')  OutDataTypeStr=uint8
  Constant3 : Constant  Value=hex2dec('bb')  OutDataTypeStr=uint8
  Constant4 : Constant  Value=0  OutDataTypeStr=single
  Constant5 : Constant  Value=0.5  OutDataTypeStr=single
  Constant6 : Constant  Value=0  OutDataTypeStr=single
  Constant7 : Constant  Value=0  OutDataTypeStr=uint8
  Constant8 : Constant  OutDataTypeStr=uint8
  Data Store Memory18 : DataStoreMemory  DataStoreName=spiTx  ReadBeforeWriteMsg=warning  WriteAfterWriteMsg=warning  WriteAfterReadMsg=warning  InitialValue=zeros(1,192)  ShowAdditionalParam=off  OutDataTypeStr=uint8
  Data Store Memory19 : DataStoreMemory  DataStoreName=BattVolt  ReadBeforeWriteMsg=warning  WriteAfterWriteMsg=warning  WriteAfterReadMsg=warning  InitialValue=[0]  ShowAdditionalParam=off  OutDataTypeStr=uint16
  Data Store Memory20 : DataStoreMemory  DataStoreName=IgnState  ReadBeforeWriteMsg=warning  WriteAfterWriteMsg=warning  WriteAfterReadMsg=warning  InitialValue=[170]  ShowAdditionalParam=off  OutDataTypeStr=uint8
  Data Store Read : DataStoreRead  DataStoreName=BuzzerBool
  Data Store Read1 : DataStoreRead  DataStoreName=spiMsg7
  Data Store Read10 : DataStoreRead  DataStoreName=spiMsg6
  Data Store Read11 : DataStoreRead  DataStoreName=spiMsg0
  Data Store Read12 : DataStoreRead  DataStoreName=spiMsg8
  Data Store Read13 : DataStoreRead  DataStoreName=spiMsg9
  Data Store Read14 : DataStoreRead  DataStoreName=spiMsg10
  Data Store Read15 : DataStoreRead  DataStoreName=spiMsg11
  Data Store Read16 : DataStoreRead  DataStoreName=spiMsg12
  Data Store Read17 : DataStoreRead  DataStoreName=spiMsg13
  Data Store Read18 : DataStoreRead  DataStoreName=spiMsg23
  Data Store Read19 : DataStoreRead  DataStoreName=spiMsg22
  Data Store Read2 : DataStoreRead  DataStoreName=spiTx
  Data Store Read20 : DataStoreRead  DataStoreName=spiMsg16
  Data Store Read21 : DataStoreRead  DataStoreName=spiMsg17
  Data Store Read22 : DataStoreRead  DataStoreName=spiMsg18
  Data Store Read23 : DataStoreRead  DataStoreName=spiMsg19
  Data Store Read24 : DataStoreRead  DataStoreName=spiMsg20
  Data Store Read25 : DataStoreRead  DataStoreName=spiMsg21
  Data Store Read3 : DataStoreRead  DataStoreName=spiMsg15
  Data Store Read4 : DataStoreRead  DataStoreName=spiMsg14
  Data Store Read5 : DataStoreRead  DataStoreName=spiMsg1
  Data Store Read6 : DataStoreRead  DataStoreName=spiMsg2
  Data Store Read7 : DataStoreRead  DataStoreName=spiMsg3
  Data Store Read8 : DataStoreRead  DataStoreName=spiMsg4
  Data Store Read9 : DataStoreRead  DataStoreName=spiMsg5
  Data Store Write : DataStoreWrite  DataStoreName=BattVolt
  Data Store Write1 : DataStoreWrite  DataStoreName=spiTx
  Data Store Write10 : DataStoreWrite  DataStoreName=spiRx7
  Data Store Write11 : DataStoreWrite  DataStoreName=spiRx15
  Data Store Write12 : DataStoreWrite  DataStoreName=spiMsg8
  Data Store Write13 : DataStoreWrite  DataStoreName=spiMsg9
  Data Store Write14 : DataStoreWrite  DataStoreName=spiRx10
  Data Store Write15 : DataStoreWrite  DataStoreName=spiRx11
  Data Store Write16 : DataStoreWrite  DataStoreName=spiRx12
  Data Store Write17 : DataStoreWrite  DataStoreName=spiRx13
  Data Store Write18 : DataStoreWrite  DataStoreName=spiRx14
  Data Store Write19 : DataStoreWrite  DataStoreName=spiRx23
  Data Store Write2 : DataStoreWrite  DataStoreName=spiRx0
  Data Store Write20 : DataStoreWrite  DataStoreName=spiMsg16
  Data Store Write21 : DataStoreWrite  DataStoreName=spiMsg17
  Data Store Write22 : DataStoreWrite  DataStoreName=spiRx18
  Data Store Write23 : DataStoreWrite  DataStoreName=spiRx19
  Data Store Write24 : DataStoreWrite  DataStoreName=spiRx20
  Data Store Write25 : DataStoreWrite  DataStoreName=spiRx21
  Data Store Write26 : DataStoreWrite  DataStoreName=spiRx22
  Data Store Write3 : DataStoreWrite  DataStoreName=IgnState
  Data Store Write4 : DataStoreWrite  DataStoreName=spiRx1
  Data Store Write5 : DataStoreWrite  DataStoreName=spiRx2
  Data Store Write6 : DataStoreWrite  DataStoreName=spiRx3
  Data Store Write7 : DataStoreWrite  DataStoreName=spiRx4
  Data Store Write8 : DataStoreWrite  DataStoreName=spiRx5
  Data Store Write9 : DataStoreWrite  DataStoreName=spiRx6
  Delay : Delay  DelayLength=1  InitialCondition=0
  Demux : Demux  Outputs=24
  Digital_Input : mbd_s32k1xx_ec_toolbox/GPIO Blocks/Digital_Input  gpio_pin=PTE13: [PTE13 | Port E I/O]  pull_resistor=Pulldown  passive_filter=off
  Digital_Output2 : mbd_s32k1xx_ec_toolbox/GPIO Blocks/Digital_Output  gpio_pin=PTD7: [PTD7 | Port D I/O]  init_val=High  drive_strength=Low
  Extract Bits : simulink/Logic and Bit Operations/Extract Bits  bitsToExtract=Lower half  numBits=8  bitIdxRange=[0 7]  outScalingMode=Treat bit field as an integer
  FTM_PWM_Config : mbd_s32k1xx_ec_toolbox/Motor Control Blocks/FTM Blocks/FTM_PWM_Config  ftmModule=2  ftmMode=Edge-Aligned PWM  ftmSourceClock=80 MHz  swcontrol_enable=off  chan0En=off  chan0Type=Complementary  chan2En=on  chan2Type=Independent  chan4En=off  chan4Type=Independent  chan6En=off  chan6Type=Independent  ftmPwmUnits=Hz  outFrequency=4000  ftmPeriod=20000  ftmPrescaler=Divide by 1  deadtimeUnits=Nanoseconds  deadtimeNs=0  deadtimeTicks=0  deadtimePrescaler=Divide by 1  dutyCycleCh0=0.25  dutyCycleCh1=0.25  dutyCycleCh2=0  dutyCycleCh3=0.5  dutyCycleCh4=0.25  dutyCycleCh5=0.25  dutyCycleCh6=0.25  dutyCycleCh7=0.25  dutyCycleSim=off  startAfterInit=on  showAdvOpt=on  pinFtmCh0=PTC5: [FTM2_CH0 | FTM Channel]  pinFtmCh1=None  pinPolCh0=Active Low  pinPolCh1=Active Low  outputComplem0=Main duplicated  outputLevel0=Low  outputLevel1=Low  pinFtmCh2=PTE4: [FTM2_CH2 | FTM Channel]  pinFtmCh3=PTD5: [FTM2_CH3 | FTM Channel]  pinPolCh2=Active Low  pinPolCh3=Active High  outputComplem2=Main duplicated  outputLevel2=High  outputLevel3=Low  pinFtmCh4=PTD13: [FTM2_CH4 | FTM Channel]  pinFtmCh5=None  pinPolCh4=Active Low  pinPolCh5=Active Low  outputComplem4=Main duplicated  outputLevel4=Low  outputLevel5=Low  pinFtmCh6=PTC12: [FTM2_CH6 | FTM Channel]  pinFtmCh7=None  pinPolCh6=Active Low  pinPolCh7=Active Low  outputComplem6=Main duplicated  outputLevel6=Low  outputLevel7=Low  initTrigger=off  chTrigger0=off  chTrigger1=off  chTrigger2=off  chTrigger3=off  chTrigger4=off  chTrigger5=off  chTrigger6=off  chTrigger7=off  mcuTargetUpdate=on  pwmSyncTrg=Software trigger  pwmSyncHwRouting=TRGMUX_FTM7  pwmSyncTrg0=off  pwmSyncTrg1=off  pwmSyncTrg2=off  pwmSyncAutoClear=on  pwmSyncMinLoad=on  pwmSyncMaxLoad=on  pwmSyncInvert=System Clock  pwmSyncOutControl=System Clock  pwmSyncOutMask=System Clock  pwmSyncCounterInitial=System Clock  pwmSyncPoints=Update now  reloadEnable=off  reloadPriority=15  reloadHalfCycle=off  reloadHCR=0  reloadFrequency=0  chnMatch0=off  chnMatch1=off  chnMatch2=off  chnMatch3=off  chnMatch4=off  chnMatch5=off  chnMatch6=off  chnMatch7=off  pwmFaultProtection=off  pwmFaultInterrupt=off  pwmFaultClearing=Fault control disabled  pwmFaultPinState=Safe Value  pwmFaultFilterValue=0  pwmFaultPriority=15  fault_disen_0=off  fault_filter_0=off  fault_polarity_0=Active High  fault_disen_1=off  fault_filter_1=off  fault_polarity_1=Active high  fault_disen_2=off  fault_filter_2=off  fault_polarity_2=Active high  fault_disen_3=off  fault_filter_3=off  fault_polarity_3=Active high  fault_pin_0=None  fault_pin_1=None  fault_pin_2=None  fault_pin_3=None
  Gain : Gain  Gain=9.5  OutDataTypeStr=uint16
  LPSPI_Slave_Transfer : mbd_s32k1xx_ec_toolbox/Communication Blocks/SPI Blocks/LPSPI_Slave_Transfer  instance=1  pcs=3  pcs_polarity=ActiveLow  xfermode=Non blocking  timeout=70  spi_upd=on
  Mux : Mux  Inputs=24
  Relational Operator : RelationalOperator  Operator=<  OutDataTypeStr=boolean  RndMeth=Simplest  InputSameDT=on
  Shutdown Delay (s) : Constant  Value=20  OutDataTypeStr=uint32
  Sum : Sum
  Switch : Switch  Criteria=u2 > Threshold
  Switch1 : Switch  Criteria=u2 > Threshold  OutDataTypeStr=single
  Switch2 : Switch  Criteria=u2 > Threshold  OutDataTypeStr=uint32
  WDOG_Trigger : mbd_s32k1xx_ec_toolbox/Core and System Blocks/WDOG Blocks/WDOG_Trigger
  Weighted Sample Time : SampleTimeMath  TsampMathOp=/  OutDataTypeStr=Inherit: Inherit via back propagation  RndMeth=Round  SaturateOnIntegerOverflow=on
  wires:
  Constant3/1 -> Switch/3
  Constant2/1 -> Switch/1
  Extract Bits/1 -> Gain/1
  ADC_Start/1 -> Extract Bits/1
  Switch/1 -> Data Store Write3/1
  Digital_Input/1 -> Switch2/2, Switch/2  "Ignition"
  Data Store Read/1 -> Switch1/2  "On/off"
  Switch1/1 -> FTM_PWM_Config/2
  Constant5/1 -> Switch1/1
  Constant4/1 -> FTM_PWM_Config/1
  Constant6/1 -> Switch1/3
  Gain/1 -> Data Store Write/1
  LPSPI_Slave_Transfer/1 -> Demux/1
  Data Store Read5/1 -> Mux/2
  Data Store Read1/1 -> Mux/8
  Data Store Read10/1 -> Mux/7
  Demux/2 -> Data Store Write4/1
  Demux/5 -> Data Store Write7/1
  Data Store Read8/1 -> Mux/5
  Data Store Read6/1 -> Mux/3
  Data Store Read9/1 -> Mux/6
  Data Store Read7/1 -> Mux/4
  Demux/3 -> Data Store Write5/1
  Demux/4 -> Data Store Write6/1
  Demux/1 -> Data Store Write2/1
  Demux/6 -> Data Store Write8/1
  Demux/7 -> Data Store Write9/1
  Demux/8 -> Data Store Write10/1
  Mux/1 -> Data Store Write1/1
  Data Store Read2/1 -> LPSPI_Slave_Transfer/1
  Weighted Sample Time/1 -> Relational Operator/2
  Switch2/1 -> Delay/1, Relational Operator/1
  Constant7/1 -> Switch2/1
  Shutdown Delay (s)/1 -> Weighted Sample Time/1
  Constant8/1 -> Sum/1
  Relational Operator/1 -> Digital_Output2/1
  Delay/1 -> Sum/2
  Sum/1 -> Switch2/3
  Data Store Read11/1 -> Mux/1
  Data Store Read14/1 -> Mux/11
  Data Store Read13/1 -> Mux/10
  Data Store Read12/1 -> Mux/9
  Data Store Read3/1 -> Mux/16
  Data Store Read16/1 -> Mux/13
  Data Store Read17/1 -> Mux/14
  Data Store Read15/1 -> Mux/12
  Data Store Read4/1 -> Mux/15
  Data Store Read22/1 -> Mux/19
  Data Store Read21/1 -> Mux/18
  Data Store Read20/1 -> Mux/17
  Data Store Read18/1 -> Mux/24
  Data Store Read24/1 -> Mux/21
  Data Store Read25/1 -> Mux/22
  Data Store Read23/1 -> Mux/20
  Data Store Read19/1 -> Mux/23
  Demux/9 -> Data Store Write12/1
  Demux/10 -> Data Store Write13/1
  Demux/11 -> Data Store Write14/1
  Demux/12 -> Data Store Write15/1
  Demux/13 -> Data Store Write16/1
  Demux/14 -> Data Store Write17/1
  Demux/15 -> Data Store Write18/1
  Demux/16 -> Data Store Write11/1
  Demux/17 -> Data Store Write20/1
  Demux/18 -> Data Store Write21/1
  Demux/19 -> Data Store Write22/1
  Demux/20 -> Data Store Write23/1
  Demux/21 -> Data Store Write24/1
  Demux/22 -> Data Store Write25/1
  Demux/23 -> Data Store Write26/1
  Demux/24 -> Data Store Write19/1
